simulink model "fft_biplex_test3"  (Simulink 7.6)
settings: Solver=ode45  StartTime=0.0  StopTime=5000  RelTol=1e-3
libraries: xbsIndex_r4 x1382, casper_library x82, monroe_library x27, xps_library x17, dspsigops x16, simulink x1
(part 5 of 13)

== system fft_biplex_test3/FFT_Biplex_4x/biplex_muxsel_gen/coeff_gen7 ==
  sync : Inport
  Concat : xbsIndex_r4/Concat  num_inputs=2  dbl_ovrd=off  block_type=concat
  Concat1 : xbsIndex_r4/Concat  num_inputs=2  dbl_ovrd=off  block_type=concat
  Concat2 : xbsIndex_r4/Concat  num_inputs=2  dbl_ovrd=off  block_type=concat
  Constant : xbsIndex_r4/Constant  arith_type=Boolean  const=0  n_bits=16  bin_pt=14  explicit_period=on  period=1  equ=P=C  opselect=C  inp2=PCIN>>17  opr=+  inp1=P  carry=CIN  dbl_ovrd=off  block_type=constant
  Constant1 : xbsIndex_r4/Constant  arith_type=Boolean  const=1  n_bits=16  bin_pt=14  explicit_period=off  period=1  equ=P=C  opselect=C  inp2=PCIN>>17  opr=+  inp1=P  carry=CIN  dbl_ovrd=off  block_type=constant
  Constant3 : xbsIndex_r4/Constant  arith_type=Signed (2's comp)  const=0  n_bits=18  bin_pt=17  explicit_period=on  period=1  equ=P=C  opselect=C  inp2=PCIN>>17  opr=+  inp1=P  carry=CIN  dbl_ovrd=off  block_type=constant
  Constant4 : xbsIndex_r4/Constant  arith_type=Boolean  const=0  n_bits=16  bin_pt=14  explicit_period=off  period=1  equ=P=C  opselect=C  inp2=PCIN>>17  opr=+  inp1=P  carry=CIN  dbl_ovrd=off  block_type=constant
  Constant5 : xbsIndex_r4/Constant  arith_type=Unsigned  const=2  n_bits=9  bin_pt=0  explicit_period=on  period=1  equ=P=C  opselect=C  inp2=PCIN>>17  opr=+  inp1=P  carry=CIN  dbl_ovrd=off  block_type=constant
  Counter : xbsIndex_r4/Counter  cnt_type=Free Running  cnt_to=Inf  operation=Up  start_count=0  cnt_by_val=1  arith_type=Unsigned  n_bits=9  bin_pt=0  load_pin=on  rst=off  en=off  explicit_period=on  period=1  dbl_ovrd=off  use_behavioral_HDL=off  implementation=Fabric  block_type=counter
  Delay : xbsIndex_r4/Delay  en=off  latency=0  dbl_ovrd=off  reg_retiming=off  block_type=delay
  Dual Port RAM4 : xbsIndex_r4/Dual Port RAM  depth=128  initVector=[0 -1 -0.707106781186547 -0.707106781186548 -0.38268343236509 -0.923879532511287 -0.923879532511287 -0.38268343236509 -0.195090322016128 -0.98078528040323 -0.831469612302545 -0.555570233019602 -0.555570233019602 -0.831469612302545 -0.98078528040323 -0.195090322016129 -0.0980171403295606 -0.995184726672197 -0.773010453362737 -0.634393284163645 -0.471396736825998 -0.881921264348355 -0.956940335732209 -0.290284677254462 -0.290284677254462 -0.956940335732209 -0.881921264348355 -0.471396736825998 -0.634393284163645 -0.773010453362737 -0.995184726672197 -0.0980171403295608 -0.049067674327418 -0.998795456205172 -0.740951125354959 -0.671558954847019 -0.427555093430282 -0.903989293123443 -0.941544065183021 -0.33688985339222 -0.242980179903264 -0.970031253194544 -0.857728610000272 -0.514102744193222 -0.595699304492433 -0.803207531480645 -0.989176509964781 -0.146730474455362 -0.146730474455362 -0.989176509964781 -0.803207531480645 -0.595699304492433 -0.514102744193222 -0.857728610000272 -0.970031253194544 -0.242980179903264 -0.33688985339222 -0.941544065183021 -0.903989293123443 -0.427555093430282 -0.671558954847018 -0.740951125354959 -0.998795456205172 -0.049067674327418 1 6.12323399573677e-17 0.707106781186548 -0.707106781186547 0.923879532511287 -0.38268343236509 0.38268343236509 -0.923879532511287 0.98078528040323 -0.195090322016128 0.555570233019602 -0.831469612302545 0.831469612302545 -0.555570233019602 0.195090322016128 -0.98078528040323 0.995184726672197 -0.0980171403295606 0.634393284163645 -0.773010453362737 0.881921264348355 -0.471396736825998 0.290284677254462 -0.956940335732209 0.956940335732209 -0.290284677254462 0.471396736825998 -0.881921264348355 0.773010453362737 -0.634393284163645 0.0980171403295608 -0.995184726672197 0.998795456205172 -0.049067674327418 0.671558954847018 -0.740951125354959 0.903989293123443 -0.427555093430282 0.33688985339222 -0.941544065183021 0.970031253194544 -0.242980179903264 0.514102744193222 -0.857728610000272 0.803207531480645 -0.595699304492433 0.146730474455362 -0.989176509964781 0.989176509964781 -0.146730474455362 0.595699304492433 -0.803207531480645 0.857728610000272 -0.514102744193222 0.242980179903264 -0.970031253194544 0.941544065183021 -0.33688985339222 0.427555093430282 -0.903989293123443 0.740951125354959 -0.671558954847018 0.0490676743274181 -0.998795456205172]  distributed_mem=Block RAM  init_a=0  init_b=0  rst_a=off  rst_b=off  en_a=off  en_b=off  latency=2  write_mode_A=No Read On Write  write_mode_B=No Read On Write  dbl_ovrd=off  optimize=Area  use_rpm=on  block_type=dpram
  Reinterpret : xbsIndex_r4/Reinterpret  force_arith_type=on  arith_type=Unsigned  force_bin_pt=on  bin_pt=0  block_type=reinterpret
      settings: infoedit="Changes signal type without altering the binary representation.   You can changed the signal between signed and unsigned, and relocate the binary point.<br><br>Hardware notes: In hardware this block costs nothing.<br><br>Example:  Suppose the input is 6 bits wide, signed, with 2 fractional bits, and the output is forced to unsigned with 0 fractional bits.  Then an input of -2.0 (1110.00 in binary 2's complement) becomes an output of 56 (111000 in binary)."
  Reinterpret1 : xbsIndex_r4/Reinterpret  force_arith_type=on  arith_type=Unsigned  force_bin_pt=on  bin_pt=0  block_type=reinterpret
      settings: infoedit="Changes signal type without altering the binary representation.   You can changed the signal between signed and unsigned, and relocate the binary point.<br><br>Hardware notes: In hardware this block costs nothing.<br><br>Example:  Suppose the input is 6 bits wide, signed, with 2 fractional bits, and the output is forced to unsigned with 0 fractional bits.  Then an input of -2.0 (1110.00 in binary 2's complement) becomes an output of 56 (111000 in binary)."
  count_slice : xbsIndex_r4/Slice  nbits=6  boolean_output=off  mode=Upper Bit Location + Width  bit1=0  base1=MSB of Input  bit0=0  base0=MSB of Input  dbl_ovrd=off  block_type=slice
  coeff : Outport
  wires:
  Constant1/1 -> Concat/1  "xlsub2_Constant1_out1"
  Constant4/1 -> Concat1/1  "xlsub2_Constant4_out1"
  sync/1 -> Counter/1
  Constant5/1 -> Counter/2  "xlsub2_Constant5_out1"
  Counter/1 -> count_slice/1
  Concat2/1 -> Delay/1  "xlsub2_Concat2_out1"
  Delay/1 -> coeff/1
  Concat/1 -> Dual Port RAM4/1  "xlsub2_Concat_out1"
  Concat1/1 -> Dual Port RAM4/4  "xlsub2_Concat1_out1"
  Dual Port RAM4/1 -> Reinterpret/1  "xlsub2_Dual_Port_RAM4_out1"
  Reinterpret/1 -> Concat2/1  "xlsub2_Reinterpret_out1"
  Dual Port RAM4/2 -> Reinterpret1/1  "xlsub2_Dual_Port_RAM4_out2"
  Reinterpret1/1 -> Concat2/2  "xlsub2_Reinterpret1_out1"
  Constant/1 -> Dual Port RAM4/3, Dual Port RAM4/6  "xlsub2_Constant_out1"
  Constant3/1 -> Dual Port RAM4/2, Dual Port RAM4/5  "xlsub2_Constant3_out1"
  count_slice/1 -> Concat/2, Concat1/2  "xlsub2_Counter_out1"

== system fft_biplex_test3/FFT_Biplex_4x/biplex_muxsel_gen/coeff_gen8 ==
  sync : Inport
  Concat : xbsIndex_r4/Concat  num_inputs=2  dbl_ovrd=off  block_type=concat
  Concat1 : xbsIndex_r4/Concat  num_inputs=2  dbl_ovrd=off  block_type=concat
  Concat2 : xbsIndex_r4/Concat  num_inputs=2  dbl_ovrd=off  block_type=concat
  Constant : xbsIndex_r4/Constant  arith_type=Boolean  const=0  n_bits=16  bin_pt=14  explicit_period=on  period=1  equ=P=C  opselect=C  inp2=PCIN>>17  opr=+  inp1=P  carry=CIN  dbl_ovrd=off  block_type=constant
  Constant1 : xbsIndex_r4/Constant  arith_type=Boolean  const=1  n_bits=16  bin_pt=14  explicit_period=off  period=1  equ=P=C  opselect=C  inp2=PCIN>>17  opr=+  inp1=P  carry=CIN  dbl_ovrd=off  block_type=constant
  Constant3 : xbsIndex_r4/Constant  arith_type=Signed (2's comp)  const=0  n_bits=18  bin_pt=17  explicit_period=on  period=1  equ=P=C  opselect=C  inp2=PCIN>>17  opr=+  inp1=P  carry=CIN  dbl_ovrd=off  block_type=constant
  Constant4 : xbsIndex_r4/Constant  arith_type=Boolean  const=0  n_bits=16  bin_pt=14  explicit_period=off  period=1  equ=P=C  opselect=C  inp2=PCIN>>17  opr=+  inp1=P  carry=CIN  dbl_ovrd=off  block_type=constant
  Constant5 : xbsIndex_r4/Constant  arith_type=Unsigned  const=2  n_bits=9  bin_pt=0  explicit_period=on  period=1  equ=P=C  opselect=C  inp2=PCIN>>17  opr=+  inp1=P  carry=CIN  dbl_ovrd=off  block_type=constant
  Counter : xbsIndex_r4/Counter  cnt_type=Free Running  cnt_to=Inf  operation=Up  start_count=0  cnt_by_val=1  arith_type=Unsigned  n_bits=9  bin_pt=0  load_pin=on  rst=off  en=off  explicit_period=on  period=1  dbl_ovrd=off  use_behavioral_HDL=off  implementation=Fabric  block_type=counter
  Delay : xbsIndex_r4/Delay  en=off  latency=0  dbl_ovrd=off  reg_retiming=off  block_type=delay
  Dual Port RAM4 : xbsIndex_r4/Dual Port RAM  depth=256  initVector=[0 -1 -0.707106781186547 -0.707106781186548 -0.38268343236509 -0.923879532511287 -0.923879532511287 -0.38268343236509 -0.195090322016128 -0.98078528040323 -0.831469612302545 -0.555570233019602 -0.555570233019602 -0.831469612302545 -0.98078528040323 -0.195090322016129 -0.0980171403295606 -0.995184726672197 -0.773010453362737 -0.634393284163645 -0.471396736825998 -0.881921264348355 -0.956940335732209 -0.290284677254462 -0.290284677254462 -0.956940335732209 -0.881921264348355 -0.471396736825998 -0.634393284163645 -0.773010453362737 -0.995184726672197 -0.0980171403295608 -0.049067674327418 -0.998795456205172 -0.740951125354959 -0.671558954847019 -0.427555093430282 -0.903989293123443 -0.941544065183021 -0.33688985339222 -0.242980179903264 -0.970031253194544 -0.857728610000272 -0.514102744193222 -0.595699304492433 -0.803207531480645 -0.989176509964781 -0.146730474455362 -0.146730474455362 -0.989176509964781 -0.803207531480645 -0.595699304492433 -0.514102744193222 -0.857728610000272 -0.970031253194544 -0.242980179903264 -0.33688985339222 -0.941544065183021 -0.903989293123443 -0.427555093430282 -0.671558954847018 -0.740951125354959 -0.998795456205172 -0.049067674327418 -0.0245412285229123 -0.999698818696204 -0.724247082951467 -0.689540544737067 -0.40524131400499 -0.914209755703531 -0.932992798834739 -0.359895036534988 -0.21910124015687 -0.975702130038529 -0.844853565249707 -0.534997619887097 -0.575808191417845 -0.817584813151584 -0.985277642388941 -0.170961888760301 -0.122410675199216 -0.99247953459871 -0.788346427626606 -0.615231590580627 -0.492898192229784 -0.870086991108711 -0.96377606579544 -0.266712757474898 -0.313681740398892 -0.949528180593037 -0.893224301195515 -0.449611329654607 -0.653172842953777 -0.757208846506485 -0.99729045667869 -0.0735645635996677 -0.0735645635996674 -0.99729045667869 -0.757208846506485 -0.653172842953777 -0.449611329654607 -0.893224301195515 -0.949528180593037 -0.313681740398891 -0.266712757474898 -0.96377606579544 -0.870086991108711 -0.492898192229784 -0.615231590580627 -0.788346427626606 -0.99247953459871 -0.122410675199216 -0.170961888760301 -0.985277642388941 -0.817584813151584 -0.575808191417845 -0.534997619887097 -0.844853565249707 -0.975702130038529 -0.21910124015687 -0.359895036534988 -0.932992798834739 -0.914209755703531 -0.40524131400499 -0.689540544737067 -0.724247082951467 -0.999698818696204 -0.0245412285229123 1 6.12323399573677e-17 0.707106781186548 -0.707106781186547 0.923879532511287 -0.38268343236509 0.38268343236509 -0.923879532511287 0.98078528040323 -0.195090322016128 0.555570233019602 -0.831469612302545 0.831469612302545 -0.555570233019602 0.195090322016128 -0.98078528040323 0.995184726672197 -0.0980171403295606 0.634393284163645 -0.773010453362737 0.881921264348355 -0.471396736825998 0.290284677254462 -0.956940335732209 0.956940335732209 -0.290284677254462 0.471396736825998 -0.881921264348355 0.773010453362737 -0.634393284163645 0.0980171403295608 -0.995184726672197 0.998795456205172 -0.049067674327418 0.671558954847018 -0.740951125354959 0.903989293123443 -0.427555093430282 0.33688985339222 -0.941544065183021 0.970031253194544 -0.242980179903264 0.514102744193222 -0.857728610000272 0.803207531480645 -0.595699304492433 0.146730474455362 -0.989176509964781 0.989176509964781 -0.146730474455362 0.595699304492433 -0.803207531480645 0.857728610000272 -0.514102744193222 0.242980179903264 -0.970031253194544 0.941544065183021 -0.33688985339222 0.427555093430282 -0.903989293123443 0.740951125354959 -0.671558954847018 0.0490676743274181 -0.998795456205172 0.999698818696204 -0.0245412285229121 0.689540544737067 -0.724247082951467 0.914209755703531 -0.40524131400499 0.359895036534988 -0.932992798834739 0.975702130038529 -0.21910124015687 0.534997619887097 -0.844853565249707 0.817584813151584 -0.575808191417845 0.170961888760301 -0.985277642388941 0.99247953459871 -0.122410675199216 0.615231590580627 -0.788346427626606 0.870086991108711 -0.492898192229784 0.266712757474898 -0.96377606579544 ...(+737 chars)]  distributed_mem=Block RAM  init_a=0  init_b=0  rst_a=off  rst_b=off  en_a=off  en_b=off  latency=2  write_mode_A=No Read On Write  write_mode_B=No Read On Write  dbl_ovrd=off  optimize=Area  use_rpm=on  block_type=dpram
  Reinterpret : xbsIndex_r4/Reinterpret  force_arith_type=on  arith_type=Unsigned  force_bin_pt=on  bin_pt=0  block_type=reinterpret
      settings: infoedit="Changes signal type without altering the binary representation.   You can changed the signal between signed and unsigned, and relocate the binary point.<br><br>Hardware notes: In hardware this block costs nothing.<br><br>Example:  Suppose the input is 6 bits wide, signed, with 2 fractional bits, and the output is forced to unsigned with 0 fractional bits.  Then an input of -2.0 (1110.00 in binary 2's complement) becomes an output of 56 (111000 in binary)."
  Reinterpret1 : xbsIndex_r4/Reinterpret  force_arith_type=on  arith_type=Unsigned  force_bin_pt=on  bin_pt=0  block_type=reinterpret
      settings: infoedit="Changes signal type without altering the binary representation.   You can changed the signal between signed and unsigned, and relocate the binary point.<br><br>Hardware notes: In hardware this block costs nothing.<br><br>Example:  Suppose the input is 6 bits wide, signed, with 2 fractional bits, and the output is forced to unsigned with 0 fractional bits.  Then an input of -2.0 (1110.00 in binary 2's complement) becomes an output of 56 (111000 in binary)."
  count_slice : xbsIndex_r4/Slice  nbits=7  boolean_output=off  mode=Upper Bit Location + Width  bit1=0  base1=MSB of Input  bit0=0  base0=MSB of Input  dbl_ovrd=off  block_type=slice
  coeff : Outport
  wires:
  Constant1/1 -> Concat/1  "xlsub2_Constant1_out1"
  Constant4/1 -> Concat1/1  "xlsub2_Constant4_out1"
  sync/1 -> Counter/1
  Constant5/1 -> Counter/2  "xlsub2_Constant5_out1"
  Counter/1 -> count_slice/1
  Concat2/1 -> Delay/1  "xlsub2_Concat2_out1"
  Delay/1 -> coeff/1
  Concat/1 -> Dual Port RAM4/1  "xlsub2_Concat_out1"
  Concat1/1 -> Dual Port RAM4/4  "xlsub2_Concat1_out1"
  Dual Port RAM4/1 -> Reinterpret/1  "xlsub2_Dual_Port_RAM4_out1"
  Reinterpret/1 -> Concat2/1  "xlsub2_Reinterpret_out1"
  Dual Port RAM4/2 -> Reinterpret1/1  "xlsub2_Dual_Port_RAM4_out2"
  Reinterpret1/1 -> Concat2/2  "xlsub2_Reinterpret1_out1"
  Constant/1 -> Dual Port RAM4/3, Dual Port RAM4/6  "xlsub2_Constant_out1"
  Constant3/1 -> Dual Port RAM4/2, Dual Port RAM4/5  "xlsub2_Constant3_out1"
  count_slice/1 -> Concat/2, Concat1/2  "xlsub2_Counter_out1"

== system fft_biplex_test3/FFT_Biplex_4x/biplex_muxsel_gen/coeff_gen9 ==
  sync : Inport
  Concat : xbsIndex_r4/Concat  num_inputs=2  dbl_ovrd=off  block_type=concat
  Concat1 : xbsIndex_r4/Concat  num_inputs=2  dbl_ovrd=off  block_type=concat
  Concat2 : xbsIndex_r4/Concat  num_inputs=2  dbl_ovrd=off  block_type=concat
  Constant : xbsIndex_r4/Constant  arith_type=Boolean  const=0  n_bits=16  bin_pt=14  explicit_period=on  period=1  equ=P=C  opselect=C  inp2=PCIN>>17  opr=+  inp1=P  carry=CIN  dbl_ovrd=off  block_type=constant
  Constant1 : xbsIndex_r4/Constant  arith_type=Boolean  const=1  n_bits=16  bin_pt=14  explicit_period=off  period=1  equ=P=C  opselect=C  inp2=PCIN>>17  opr=+  inp1=P  carry=CIN  dbl_ovrd=off  block_type=constant
  Constant3 : xbsIndex_r4/Constant  arith_type=Signed (2's comp)  const=0  n_bits=18  bin_pt=17  explicit_period=on  period=1  equ=P=C  opselect=C  inp2=PCIN>>17  opr=+  inp1=P  carry=CIN  dbl_ovrd=off  block_type=constant
  Constant4 : xbsIndex_r4/Constant  arith_type=Boolean  const=0  n_bits=16  bin_pt=14  explicit_period=off  period=1  equ=P=C  opselect=C  inp2=PCIN>>17  opr=+  inp1=P  carry=CIN  dbl_ovrd=off  block_type=constant
  Constant5 : xbsIndex_r4/Constant  arith_type=Unsigned  const=2  n_bits=9  bin_pt=0  explicit_period=on  period=1  equ=P=C  opselect=C  inp2=PCIN>>17  opr=+  inp1=P  carry=CIN  dbl_ovrd=off  block_type=constant
  Counter : xbsIndex_r4/Counter  cnt_type=Free Running  cnt_to=Inf  operation=Up  start_count=0  cnt_by_val=1  arith_type=Unsigned  n_bits=9  bin_pt=0  load_pin=on  rst=off  en=off  explicit_period=on  period=1  dbl_ovrd=off  use_behavioral_HDL=off  implementation=Fabric  block_type=counter
  Delay : xbsIndex_r4/Delay  en=off  latency=0  dbl_ovrd=off  reg_retiming=off  block_type=delay
  Dual Port RAM4 : xbsIndex_r4/Dual Port RAM  depth=512  initVector=[0 -1 -0.707106781186547 -0.707106781186548 -0.38268343236509 -0.923879532511287 -0.923879532511287 -0.38268343236509 -0.195090322016128 -0.98078528040323 -0.831469612302545 -0.555570233019602 -0.555570233019602 -0.831469612302545 -0.98078528040323 -0.195090322016129 -0.0980171403295606 -0.995184726672197 -0.773010453362737 -0.634393284163645 -0.471396736825998 -0.881921264348355 -0.956940335732209 -0.290284677254462 -0.290284677254462 -0.956940335732209 -0.881921264348355 -0.471396736825998 -0.634393284163645 -0.773010453362737 -0.995184726672197 -0.0980171403295608 -0.049067674327418 -0.998795456205172 -0.740951125354959 -0.671558954847019 -0.427555093430282 -0.903989293123443 -0.941544065183021 -0.33688985339222 -0.242980179903264 -0.970031253194544 -0.857728610000272 -0.514102744193222 -0.595699304492433 -0.803207531480645 -0.989176509964781 -0.146730474455362 -0.146730474455362 -0.989176509964781 -0.803207531480645 -0.595699304492433 -0.514102744193222 -0.857728610000272 -0.970031253194544 -0.242980179903264 -0.33688985339222 -0.941544065183021 -0.903989293123443 -0.427555093430282 -0.671558954847018 -0.740951125354959 -0.998795456205172 -0.049067674327418 -0.0245412285229123 -0.999698818696204 -0.724247082951467 -0.689540544737067 -0.40524131400499 -0.914209755703531 -0.932992798834739 -0.359895036534988 -0.21910124015687 -0.975702130038529 -0.844853565249707 -0.534997619887097 -0.575808191417845 -0.817584813151584 -0.985277642388941 -0.170961888760301 -0.122410675199216 -0.99247953459871 -0.788346427626606 -0.615231590580627 -0.492898192229784 -0.870086991108711 -0.96377606579544 -0.266712757474898 -0.313681740398892 -0.949528180593037 -0.893224301195515 -0.449611329654607 -0.653172842953777 -0.757208846506485 -0.99729045667869 -0.0735645635996677 -0.0735645635996674 -0.99729045667869 -0.757208846506485 -0.653172842953777 -0.449611329654607 -0.893224301195515 -0.949528180593037 -0.313681740398891 -0.266712757474898 -0.96377606579544 -0.870086991108711 -0.492898192229784 -0.615231590580627 -0.788346427626606 -0.99247953459871 -0.122410675199216 -0.170961888760301 -0.985277642388941 -0.817584813151584 -0.575808191417845 -0.534997619887097 -0.844853565249707 -0.975702130038529 -0.21910124015687 -0.359895036534988 -0.932992798834739 -0.914209755703531 -0.40524131400499 -0.689540544737067 -0.724247082951467 -0.999698818696204 -0.0245412285229123 -0.0122715382857199 -0.999924701839145 -0.715730825283819 -0.698376249408973 -0.393992040061048 -0.919113851690058 -0.928506080473216 -0.371317193951838 -0.207111376192219 -0.978317370719628 -0.838224705554838 -0.545324988422046 -0.565731810783613 -0.824589302785025 -0.983105487431216 -0.183039887955141 -0.110222207293883 -0.993906970002356 -0.780737228572094 -0.624859488142386 -0.482183772079123 -0.876070094195407 -0.960430519415566 -0.278519689385053 -0.302005949319228 -0.953306040354194 -0.887639620402854 -0.46053871095824 -0.643831542889791 -0.765167265622459 -0.996312612182778 -0.0857973123444402 -0.0613207363022086 -0.998118112900149 -0.749136394523459 -0.662415777590172 -0.438616238538528 -0.898674465693954 -0.945607325380521 -0.325310292162263 -0.254865659604515 -0.966976471044852 -0.863972856121587 -0.503538383725718 -0.605511041404326 -0.795836904608884 -0.99090263542778 -0.134580708507126 -0.158858143333861 -0.987301418157858 -0.810457198252595 -0.585797857456439 -0.524589682678469 -0.851355193105265 -0.97293995220556 -0.231058108280671 -0.348418680249435 -0.937339011912575 -0.909167983090522 -0.416429560097637 -0.680600997795453 -0.732654271672413 -0.99932238458835 -0.0368072229413588 -0.0368072229413588 -0.99932238458835 -0.732654271672413 -0.680600997795453 -0.416429560097637 -0.909167983090522 -0.937339011912575 -0.348418680249435 -0.231058108280671 -0.97293995220556 -0.851355193105265 -0.524589682678469 -0.585797857456439 -0.810457198252595 -0.987301418157858 -0.158858143333861 -0.134580708507126 -0.99090263542778 -0.795836904608884 -0.605511041404326 ...(+5548 chars)]  distributed_mem=Block RAM  init_a=0  init_b=0  rst_a=off  rst_b=off  en_a=off  en_b=off  latency=2  write_mode_A=No Read On Write  write_mode_B=No Read On Write  dbl_ovrd=off  optimize=Area  use_rpm=on  block_type=dpram
  Reinterpret : xbsIndex_r4/Reinterpret  force_arith_type=on  arith_type=Unsigned  force_bin_pt=on  bin_pt=0  block_type=reinterpret
      settings: infoedit="Changes signal type without altering the binary representation.   You can changed the signal between signed and unsigned, and relocate the binary point.<br><br>Hardware notes: In hardware this block costs nothing.<br><br>Example:  Suppose the input is 6 bits wide, signed, with 2 fractional bits, and the output is forced to unsigned with 0 fractional bits.  Then an input of -2.0 (1110.00 in binary 2's complement) becomes an output of 56 (111000 in binary)."
  Reinterpret1 : xbsIndex_r4/Reinterpret  force_arith_type=on  arith_type=Unsigned  force_bin_pt=on  bin_pt=0  block_type=reinterpret
      settings: infoedit="Changes signal type without altering the binary representation.   You can changed the signal between signed and unsigned, and relocate the binary point.<br><br>Hardware notes: In hardware this block costs nothing.<br><br>Example:  Suppose the input is 6 bits wide, signed, with 2 fractional bits, and the output is forced to unsigned with 0 fractional bits.  Then an input of -2.0 (1110.00 in binary 2's complement) becomes an output of 56 (111000 in binary)."
  count_slice : xbsIndex_r4/Slice  nbits=8  boolean_output=off  mode=Upper Bit Location + Width  bit1=0  base1=MSB of Input  bit0=0  base0=MSB of Input  dbl_ovrd=off  block_type=slice
  coeff : Outport
  wires:
  Constant1/1 -> Concat/1  "xlsub2_Constant1_out1"
  Constant4/1 -> Concat1/1  "xlsub2_Constant4_out1"
  sync/1 -> Counter/1
  Constant5/1 -> Counter/2  "xlsub2_Constant5_out1"
  Counter/1 -> count_slice/1
  Concat2/1 -> Delay/1  "xlsub2_Concat2_out1"
  Delay/1 -> coeff/1
  Concat/1 -> Dual Port RAM4/1  "xlsub2_Concat_out1"
  Concat1/1 -> Dual Port RAM4/4  "xlsub2_Concat1_out1"
  Dual Port RAM4/1 -> Reinterpret/1  "xlsub2_Dual_Port_RAM4_out1"
  Reinterpret/1 -> Concat2/1  "xlsub2_Reinterpret_out1"
  Dual Port RAM4/2 -> Reinterpret1/1  "xlsub2_Dual_Port_RAM4_out2"
  Reinterpret1/1 -> Concat2/2  "xlsub2_Reinterpret1_out1"
  Constant/1 -> Dual Port RAM4/3, Dual Port RAM4/6  "xlsub2_Constant_out1"
  Constant3/1 -> Dual Port RAM4/2, Dual Port RAM4/5  "xlsub2_Constant3_out1"
  count_slice/1 -> Concat/2, Concat1/2  "xlsub2_Counter_out1"

== system fft_biplex_test3/FFT_Biplex_4x/biplex_muxsel_gen/cram ==
  in0 : Inport
  in1 : Inport  Port=2
  in2 : Inport  Port=3
  in3 : Inport  Port=4
  in4 : Inport  Port=5
  in5 : Inport  Port=6
  in6 : Inport  Port=7
  in7 : Inport  Port=8
  concat : xbsIndex_r4/Concat  num_inputs=8  dbl_ovrd=off  block_type=concat
  reinterpret_{1..8} (8 alike) : xbsIndex_r4/Reinterpret  force_arith_type=on  arith_type=Unsigned  force_bin_pt=on  bin_pt=0  block_type=reinterpret
      settings: infoedit="Changes signal type without altering the binary representation.   You can changed the signal between signed and unsigned, and relocate the binary point.<br><br>Hardware notes: In hardware this block costs nothing.<br><br>Example:  Suppose the input is 6 bits wide, signed, with 2 fractional bits, and the output is forced to unsigned with 0 fractional bits.  Then an input of -2.0 (1110.00 in binary 2's complement) becomes an output of 56 (111000 in binary)."
  out : Outport
  wires:
  in0/1 -> reinterpret_1/1
  in1/1 -> reinterpret_2/1
  in2/1 -> reinterpret_3/1
  in3/1 -> reinterpret_4/1
  in4/1 -> reinterpret_5/1
  in5/1 -> reinterpret_6/1
  in6/1 -> reinterpret_7/1
  in7/1 -> reinterpret_8/1
  reinterpret_1/1 -> concat/1
  reinterpret_2/1 -> concat/2
  reinterpret_3/1 -> concat/3
  reinterpret_4/1 -> concat/4
  reinterpret_5/1 -> concat/5
  reinterpret_6/1 -> concat/6
  reinterpret_7/1 -> concat/7
  reinterpret_8/1 -> concat/8
  concat/1 -> out/1

== system fft_biplex_test3/adc083000x2/adc_sim/overflow_detector ==
  s0 : Inport
  s1 : Inport  Port=2
  s2 : Inport  Port=3
  s3 : Inport  Port=4
  s4 : Inport  Port=5
  s5 : Inport  Port=6
  s6 : Inport  Port=7
  s7 : Inport  Port=8
  s8 : Inport  Port=9
  s9 : Inport  Port=10
  s10 : Inport  Port=11
  s11 : Inport  Port=12
  s12 : Inport  Port=13
  s13 : Inport  Port=14
  s14 : Inport  Port=15
  s15 : Inport  Port=16
  Add : Sum  Inputs=++++++++
  of{0..7} (8 alike) : casper_library/Misc/of1  SystemSampleTime=-1  bit_num=0  n_adc_bits=8
  overflow : Outport
  wires:
  Add/1 -> overflow/1
  of7/1 -> Add/8
  s15/1 -> of7/2
  s7/1 -> of7/1
  of6/1 -> Add/7
  s14/1 -> of6/2
  s6/1 -> of6/1
  of5/1 -> Add/6
  s13/1 -> of5/2
  s5/1 -> of5/1
  of4/1 -> Add/5
  s12/1 -> of4/2
  s4/1 -> of4/1
  of3/1 -> Add/4
  s11/1 -> of3/2
  s3/1 -> of3/1
  of2/1 -> Add/3
  s10/1 -> of2/2
  s2/1 -> of2/1
  of1/1 -> Add/2
  s9/1 -> of1/2
  s1/1 -> of1/1
  of0/1 -> Add/1
  s8/1 -> of0/2
  s0/1 -> of0/1

== system fft_biplex_test3/fft_biplex_real_4x1/bi_real_unscr_4x/complex_addsub1 ==
  a : Inport
  b : Inport  Port=2
  AddSub : xbsIndex_r4/AddSub  mode=Addition  use_carryin=off  use_carryout=off  en=off  latency=add_latency  precision=Full  arith_type=Unsigned  n_bits=8  bin_pt=2  quantization=Truncate  overflow=Wrap  dbl_ovrd=off  use_behavioral_HDL=on  hw_selection=Fabric  pipelined=off  use_rpm=on  block_type=addsub
      settings: xl_area=[0, 0, 0, 0, 0, 0, 0]  block_version=9.1.01
  AddSub1 : xbsIndex_r4/AddSub  mode=Subtraction  use_carryin=off  use_carryout=off  en=off  latency=add_latency  precision=Full  arith_type=Unsigned  n_bits=8  bin_pt=2  quantization=Truncate  overflow=Wrap  dbl_ovrd=off  use_behavioral_HDL=on  hw_selection=Fabric  pipelined=off  use_rpm=on  block_type=addsub
      settings: xl_area=[0, 0, 0, 0, 0, 0, 0]  block_version=9.1.01
  AddSub2 : xbsIndex_r4/AddSub  mode=Subtraction  use_carryin=off  use_carryout=off  en=off  latency=add_latency  precision=Full  arith_type=Unsigned  n_bits=8  bin_pt=2  quantization=Truncate  overflow=Wrap  dbl_ovrd=off  use_behavioral_HDL=on  hw_selection=Fabric  pipelined=off  use_rpm=on  block_type=addsub
      settings: xl_area=[0, 0, 0, 0, 0, 0, 0]  block_version=9.1.01
  AddSub3 : xbsIndex_r4/AddSub  mode=Addition  use_carryin=off  use_carryout=off  en=off  latency=add_latency  precision=Full  arith_type=Unsigned  n_bits=8  bin_pt=2  quantization=Truncate  overflow=Wrap  dbl_ovrd=off  use_behavioral_HDL=on  hw_selection=Fabric  pipelined=off  use_rpm=on  block_type=addsub
      settings: xl_area=[0, 0, 0, 0, 0, 0, 0]  block_version=9.1.01
  Convert{,1..3} (4 alike) : xbsIndex_r4/Convert  arith_type="Signed  (2's comp)"  n_bits=BitWidth  bin_pt=BitWidth - 1  quantization=Truncate  overflow=Wrap  en=off  latency=add_latency  dbl_ovrd=off  pipeline=off  block_type=convert
      settings: xl_area=[0, 0, 0, 0, 0, 0, 0]
  Shift{,1..3} (4 alike) : xbsIndex_r4/Shift  shift_dir=Right  shift_bits=1  en=off  latency=0  precision=Full  arith_type="Signed  (2's comp)"  n_bits=8  bin_pt=2  quantization=Truncate  overflow=Wrap  dbl_ovrd=off  block_type=shift
      settings: xl_area=[0, 0, 0, 0, 0, 0, 0]  block_version=9.1.01
  c_to_ri : casper_library/Misc/c_to_ri  SystemSampleTime=-1  n_bits=BitWidth  bin_pt=BitWidth-1
      settings: AttributesFormatString=18_17 r/i
  c_to_ri1 : casper_library/Misc/c_to_ri  SystemSampleTime=-1  n_bits=BitWidth  bin_pt=BitWidth-1
      settings: AttributesFormatString=18_17 r/i
  dsp48_complex_add : Subsystem  mask{a_bit_width=BitWidth, a_bin_pt=BitWidth-2, bw_bit_width=BitWidth, bw_bin_pt=BitWidth-2}
      mask prompts: a_bit_width "'a' bit width"; a_bin_pt "'a' binary point"; bw_bit_width "'bw' bit width"; bw_bin_pt "'bw' binary point"
  ri_to_c : casper_library/Misc/ri_to_c  SystemSampleTime=-1
  ri_to_c1 : casper_library/Misc/ri_to_c  SystemSampleTime=-1
  a+b : Outport
  a-b : Outport  Port=2
  wires:
  Convert3/1 -> ri_to_c1/1
  Convert1/1 -> ri_to_c1/2
  c_to_ri/1 -> AddSub/1, AddSub1/2, dsp48_complex_add/3(bw_re)
  c_to_ri/2 -> AddSub3/1, AddSub2/1, dsp48_complex_add/2(a_im)
  c_to_ri1/1 -> AddSub/2, AddSub1/1, dsp48_complex_add/1(a_re)
  c_to_ri1/2 -> AddSub3/2, AddSub2/2, dsp48_complex_add/4(bw_im)
  Convert/1 -> ri_to_c/1
  Convert2/1 -> ri_to_c/2
  a/1 -> c_to_ri/1
  ri_to_c/1 -> a+b/1
  ri_to_c1/1 -> a-b/1
  b/1 -> c_to_ri1/1
  Shift/1 -> Convert/1
  Shift1/1 -> Convert1/1
  Shift2/1 -> Convert2/1
  Shift3/1 -> Convert3/1
  dsp48_complex_add/3(a-bw_re) -> Shift1/1
  dsp48_complex_add/4(a-bw_im) -> Shift2/1
  dsp48_complex_add/2(a+bw_im) -> Shift3/1
  dsp48_complex_add/1(a+bw_re) -> Shift/1

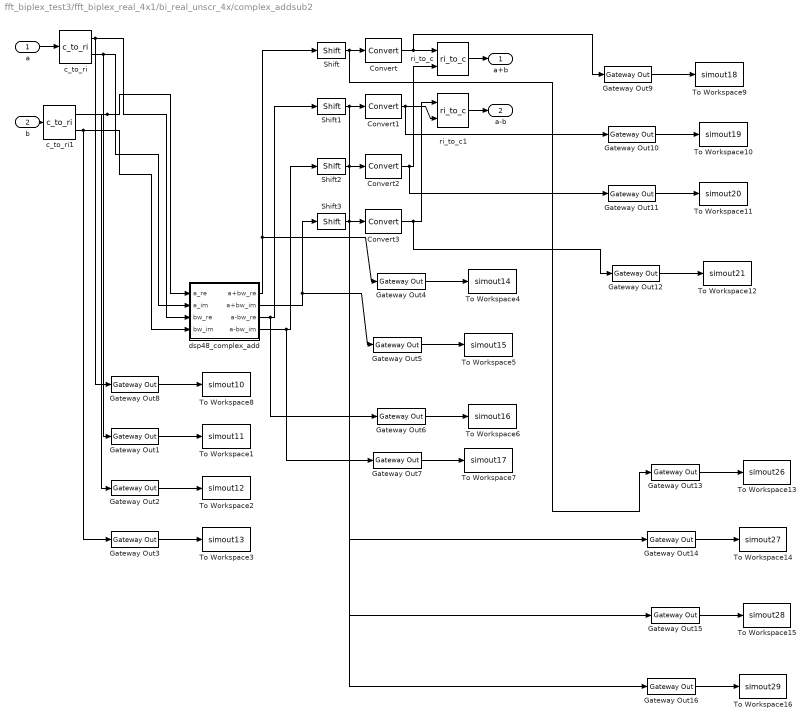
== system fft_biplex_test3/fft_biplex_real_4x1/bi_real_unscr_4x/complex_addsub2 ==
  a : Inport
  b : Inport  Port=2
  Convert{,1..3} (4 alike) : xbsIndex_r4/Convert  arith_type="Signed  (2's comp)"  n_bits=BitWidth  bin_pt=BitWidth - 1  quantization=Truncate  overflow=Wrap  en=off  latency=add_latency  dbl_ovrd=off  pipeline=off  block_type=convert
      settings: xl_area=[0, 0, 0, 0, 0, 0, 0]
  Gateway Out{1..16} (16 alike) : xbsIndex_r4/Gateway Out  hdl_port=on  timing_constraint=None  locs_specified=off  LOCs={}  block_type=gatewayout
      settings: infoedit="Gateway out block.  Converts Xilinx fixed point inputs into ouputs of type Simulink integer, double, or fixed point.<br><br>Hardware notes:  In hardware these blocks become top level output ports or are discarded, depending on how they are configured."  block_version=11.4
  Shift{,1..3} (4 alike) : xbsIndex_r4/Shift  shift_dir=Right  shift_bits=1  en=off  latency=0  precision=Full  arith_type="Signed  (2's comp)"  n_bits=8  bin_pt=2  quantization=Truncate  overflow=Wrap  dbl_ovrd=off  block_type=shift
      settings: xl_area=[0, 0, 0, 0, 0, 0, 0]  block_version=9.1.01
  To Workspace1 : ToWorkspace  VariableName=simout11  SampleTime=-1  SaveFormat=Structure
  To Workspace10 : ToWorkspace  VariableName=simout19  SampleTime=-1  SaveFormat=Structure
  To Workspace11 : ToWorkspace  VariableName=simout20  SampleTime=-1  SaveFormat=Structure
  To Workspace12 : ToWorkspace  VariableName=simout21  SampleTime=-1  SaveFormat=Structure
  To Workspace13 : ToWorkspace  VariableName=simout26  SampleTime=-1  SaveFormat=Structure
  To Workspace14 : ToWorkspace  VariableName=simout27  SampleTime=-1  SaveFormat=Structure
  To Workspace15 : ToWorkspace  VariableName=simout28  SampleTime=-1  SaveFormat=Structure
  To Workspace16 : ToWorkspace  VariableName=simout29  SampleTime=-1  SaveFormat=Structure
  To Workspace2 : ToWorkspace  VariableName=simout12  SampleTime=-1  SaveFormat=Structure
  To Workspace3 : ToWorkspace  VariableName=simout13  SampleTime=-1  SaveFormat=Structure
  To Workspace4 : ToWorkspace  VariableName=simout14  SampleTime=-1  SaveFormat=Structure
  To Workspace5 : ToWorkspace  VariableName=simout15  SampleTime=-1  SaveFormat=Structure
  To Workspace6 : ToWorkspace  VariableName=simout16  SampleTime=-1  SaveFormat=Structure
  To Workspace7 : ToWorkspace  VariableName=simout17  SampleTime=-1  SaveFormat=Structure
  To Workspace8 : ToWorkspace  VariableName=simout10  SampleTime=-1  SaveFormat=Structure
  To Workspace9 : ToWorkspace  VariableName=simout18  SampleTime=-1  SaveFormat=Structure
  c_to_ri : casper_library/Misc/c_to_ri  SystemSampleTime=-1  n_bits=BitWidth  bin_pt=BitWidth-1
      settings: AttributesFormatString=18_17 r/i
  c_to_ri1 : casper_library/Misc/c_to_ri  SystemSampleTime=-1  n_bits=BitWidth  bin_pt=BitWidth-1
      settings: AttributesFormatString=18_17 r/i
  dsp48_complex_add : Subsystem  mask{a_bit_width=BitWidth, a_bin_pt=BitWidth-2, bw_bit_width=BitWidth, bw_bin_pt=BitWidth-2}
      mask prompts: a_bit_width "'a' bit width"; a_bin_pt "'a' binary point"; bw_bit_width "'bw' bit width"; bw_bin_pt "'bw' binary point"
  ri_to_c : casper_library/Misc/ri_to_c  SystemSampleTime=-1
  ri_to_c1 : casper_library/Misc/ri_to_c  SystemSampleTime=-1
  a+b : Outport
  a-b : Outport  Port=2
  wires:
  dsp48_complex_add/1(a+bw_re) -> Shift/1, Gateway Out4/1
  dsp48_complex_add/2(a+bw_im) -> Shift3/1, Gateway Out5/1
  dsp48_complex_add/4(a-bw_im) -> Shift2/1, Gateway Out7/1
  dsp48_complex_add/3(a-bw_re) -> Shift1/1, Gateway Out6/1
  Shift3/1 -> Convert3/1, Gateway Out16/1
  Shift2/1 -> Convert2/1, Gateway Out15/1
  Shift1/1 -> Convert1/1, Gateway Out14/1
  Shift/1 -> Convert/1, Gateway Out13/1
  b/1 -> c_to_ri1/1
  ri_to_c1/1 -> a-b/1
  ri_to_c/1 -> a+b/1
  a/1 -> c_to_ri/1
  Convert2/1 -> ri_to_c/2, Gateway Out11/1
  Convert/1 -> ri_to_c/1, Gateway Out9/1
  c_to_ri1/2 -> dsp48_complex_add/4(bw_im), Gateway Out3/1
  c_to_ri1/1 -> dsp48_complex_add/1(a_re), Gateway Out2/1
  c_to_ri/2 -> dsp48_complex_add/2(a_im), Gateway Out1/1
  c_to_ri/1 -> dsp48_complex_add/3(bw_re), Gateway Out8/1
  Convert1/1 -> ri_to_c1/2, Gateway Out10/1
  Convert3/1 -> ri_to_c1/1, Gateway Out12/1
  Gateway Out8/1 -> To Workspace8/1
  Gateway Out1/1 -> To Workspace1/1
  Gateway Out2/1 -> To Workspace2/1
  Gateway Out3/1 -> To Workspace3/1
  Gateway Out4/1 -> To Workspace4/1
  Gateway Out5/1 -> To Workspace5/1
  Gateway Out6/1 -> To Workspace6/1
  Gateway Out7/1 -> To Workspace7/1
  Gateway Out9/1 -> To Workspace9/1
  Gateway Out10/1 -> To Workspace10/1
  Gateway Out11/1 -> To Workspace11/1
  Gateway Out12/1 -> To Workspace12/1
  Gateway Out13/1 -> To Workspace13/1
  Gateway Out14/1 -> To Workspace14/1
  Gateway Out15/1 -> To Workspace15/1
  Gateway Out16/1 -> To Workspace16/1

== system fft_biplex_test3/fft_biplex_real_4x1/bi_real_unscr_4x/complex_scope1 ==
  In1 : Inport
  Gateway Out15 : xbsIndex_r4/Gateway Out  hdl_port=on  timing_constraint=None  locs_specified=off  LOCs={}  block_type=gatewayout
      settings: infoedit="Gateway out block.  Converts Xilinx fixed point inputs into ouputs of type Simulink integer, double, or fixed point.<br><br>Hardware notes:  In hardware these blocks become top level output ports or are discarded, depending on how they are configured."  block_version=11.4
  Gateway Out16 : xbsIndex_r4/Gateway Out  hdl_port=on  timing_constraint=None  locs_specified=off  LOCs={}  block_type=gatewayout
      settings: infoedit="Gateway out block.  Converts Xilinx fixed point inputs into ouputs of type Simulink integer, double, or fixed point.<br><br>Hardware notes:  In hardware these blocks become top level output ports or are discarded, depending on how they are configured."  block_version=11.4
  Reinterpret : xbsIndex_r4/Reinterpret  force_arith_type=on  arith_type="Signed  (2's comp)"  force_bin_pt=on  bin_pt=17  block_type=reinterpret
      settings: infoedit="Changes signal type without altering the binary representation.   You can changed the signal between signed and unsigned, and relocate the binary point.<br><br>Hardware notes: In hardware this block costs nothing.<br><br>Example:  Suppose the input is 6 bits wide, signed, with 2 fractional bits, and the output is forced to unsigned with 0 fractional bits.  Then an input of -2.0 (1110.00 in binary 2's complement) becomes an output of 56 (111000 in binary)."
  Reinterpret1 : xbsIndex_r4/Reinterpret  force_arith_type=on  arith_type="Signed  (2's comp)"  force_bin_pt=on  bin_pt=17  block_type=reinterpret
      settings: infoedit="Changes signal type without altering the binary representation.   You can changed the signal between signed and unsigned, and relocate the binary point.<br><br>Hardware notes: In hardware this block costs nothing.<br><br>Example:  Suppose the input is 6 bits wide, signed, with 2 fractional bits, and the output is forced to unsigned with 0 fractional bits.  Then an input of -2.0 (1110.00 in binary 2's complement) becomes an output of 56 (111000 in binary)."
  c_to_ri : casper_library/Misc/c_to_ri  SystemSampleTime=-1  n_bits=18  bin_pt=17
      settings: AttributesFormatString=18_17 r/i
  Real : Outport
  Imag : Outport  Port=2
  wires:
  c_to_ri/1 -> Reinterpret/1
  c_to_ri/2 -> Reinterpret1/1
  Reinterpret/1 -> Gateway Out15/1
  Reinterpret1/1 -> Gateway Out16/1
  Gateway Out15/1 -> Real/1
  In1/1 -> c_to_ri/1
  Gateway Out16/1 -> Imag/1

== system fft_biplex_test3/fft_biplex_real_4x1/bi_real_unscr_4x/complex_scope10 ==
  In1 : Inport
  Gateway Out15 : xbsIndex_r4/Gateway Out  hdl_port=on  timing_constraint=None  locs_specified=off  LOCs={}  block_type=gatewayout
      settings: infoedit="Gateway out block.  Converts Xilinx fixed point inputs into ouputs of type Simulink integer, double, or fixed point.<br><br>Hardware notes:  In hardware these blocks become top level output ports or are discarded, depending on how they are configured."  block_version=11.4
  Gateway Out16 : xbsIndex_r4/Gateway Out  hdl_port=on  timing_constraint=None  locs_specified=off  LOCs={}  block_type=gatewayout
      settings: infoedit="Gateway out block.  Converts Xilinx fixed point inputs into ouputs of type Simulink integer, double, or fixed point.<br><br>Hardware notes:  In hardware these blocks become top level output ports or are discarded, depending on how they are configured."  block_version=11.4
  Reinterpret : xbsIndex_r4/Reinterpret  force_arith_type=on  arith_type="Signed  (2's comp)"  force_bin_pt=on  bin_pt=17  block_type=reinterpret
      settings: infoedit="Changes signal type without altering the binary representation.   You can changed the signal between signed and unsigned, and relocate the binary point.<br><br>Hardware notes: In hardware this block costs nothing.<br><br>Example:  Suppose the input is 6 bits wide, signed, with 2 fractional bits, and the output is forced to unsigned with 0 fractional bits.  Then an input of -2.0 (1110.00 in binary 2's complement) becomes an output of 56 (111000 in binary)."
  Reinterpret1 : xbsIndex_r4/Reinterpret  force_arith_type=on  arith_type="Signed  (2's comp)"  force_bin_pt=on  bin_pt=17  block_type=reinterpret
      settings: infoedit="Changes signal type without altering the binary representation.   You can changed the signal between signed and unsigned, and relocate the binary point.<br><br>Hardware notes: In hardware this block costs nothing.<br><br>Example:  Suppose the input is 6 bits wide, signed, with 2 fractional bits, and the output is forced to unsigned with 0 fractional bits.  Then an input of -2.0 (1110.00 in binary 2's complement) becomes an output of 56 (111000 in binary)."
  c_to_ri : casper_library/Misc/c_to_ri  SystemSampleTime=-1  n_bits=18  bin_pt=17
      settings: AttributesFormatString=18_17 r/i
  Real : Outport
  Imag : Outport  Port=2
  wires:
  Gateway Out16/1 -> Imag/1
  In1/1 -> c_to_ri/1
  Gateway Out15/1 -> Real/1
  Reinterpret1/1 -> Gateway Out16/1
  Reinterpret/1 -> Gateway Out15/1
  c_to_ri/2 -> Reinterpret1/1
  c_to_ri/1 -> Reinterpret/1

== system fft_biplex_test3/fft_biplex_real_4x1/bi_real_unscr_4x/complex_scope2 ==
  In1 : Inport
  Gateway Out15 : xbsIndex_r4/Gateway Out  hdl_port=on  timing_constraint=None  locs_specified=off  LOCs={}  block_type=gatewayout
      settings: infoedit="Gateway out block.  Converts Xilinx fixed point inputs into ouputs of type Simulink integer, double, or fixed point.<br><br>Hardware notes:  In hardware these blocks become top level output ports or are discarded, depending on how they are configured."  block_version=11.4
  Gateway Out16 : xbsIndex_r4/Gateway Out  hdl_port=on  timing_constraint=None  locs_specified=off  LOCs={}  block_type=gatewayout
      settings: infoedit="Gateway out block.  Converts Xilinx fixed point inputs into ouputs of type Simulink integer, double, or fixed point.<br><br>Hardware notes:  In hardware these blocks become top level output ports or are discarded, depending on how they are configured."  block_version=11.4
  Reinterpret : xbsIndex_r4/Reinterpret  force_arith_type=on  arith_type="Signed  (2's comp)"  force_bin_pt=on  bin_pt=17  block_type=reinterpret
      settings: infoedit="Changes signal type without altering the binary representation.   You can changed the signal between signed and unsigned, and relocate the binary point.<br><br>Hardware notes: In hardware this block costs nothing.<br><br>Example:  Suppose the input is 6 bits wide, signed, with 2 fractional bits, and the output is forced to unsigned with 0 fractional bits.  Then an input of -2.0 (1110.00 in binary 2's complement) becomes an output of 56 (111000 in binary)."
  Reinterpret1 : xbsIndex_r4/Reinterpret  force_arith_type=on  arith_type="Signed  (2's comp)"  force_bin_pt=on  bin_pt=17  block_type=reinterpret
      settings: infoedit="Changes signal type without altering the binary representation.   You can changed the signal between signed and unsigned, and relocate the binary point.<br><br>Hardware notes: In hardware this block costs nothing.<br><br>Example:  Suppose the input is 6 bits wide, signed, with 2 fractional bits, and the output is forced to unsigned with 0 fractional bits.  Then an input of -2.0 (1110.00 in binary 2's complement) becomes an output of 56 (111000 in binary)."
  c_to_ri : casper_library/Misc/c_to_ri  SystemSampleTime=-1  n_bits=18  bin_pt=17
      settings: AttributesFormatString=18_17 r/i
  Real : Outport
  Imag : Outport  Port=2
  wires:
  Gateway Out16/1 -> Imag/1
  In1/1 -> c_to_ri/1
  Gateway Out15/1 -> Real/1
  Reinterpret1/1 -> Gateway Out16/1
  Reinterpret/1 -> Gateway Out15/1
  c_to_ri/2 -> Reinterpret1/1
  c_to_ri/1 -> Reinterpret/1
